simulink model "Buck_Controller_Due"  (R2020a)
settings: Solver=FixedStepAuto  StartTime=0.0  StopTime=inf  FixedStep=T  RelTol=1e-3  EnableMultiTasking=on
undefined symbols (not defined in the file): ILmax, Ki_IL, Kp_IL, Kp_Uc, T, Ubat
libraries: arduinolib x8, eeStairGenerator x1
settings Model: SILPILModeSetting=veronly  ExtModeTrigDuration=2  Creator=Nguyen Tung  LastModifiedBy=Nguyen Tung
settings OptimizationCC: StrengthReduction=on  PassReuseOutputArgsAs=Individual arguments  ZeroExternalMemoryAtStartup=off  ZeroInternalMemoryAtStartup=off  MaxStackSize=64  OptimizeBlockOrder=speed  OptimizationPriority=Speed  OptimizationCustomize=off  MultiThreadedLoops=on  EfficientTunableParamExpr=on
settings DebuggingCC: ParameterTunabilityLossMsg=error
settings HardwareCC: ProdBitPerPointer=32  ProdBitPerSizeT=32  ProdBitPerPtrDiffT=32  ProdLargestAtomicInteger=Long  ProdLargestAtomicFloat=Double  ProdWordSize=32  ProdHWDeviceType=ARM Compatible->ARM Cortex
settings SFSimCC: MATLABDynamicMemAlloc=off
settings RTWCC: SystemTargetFile=ert.tlc  HardwareBoard=Arduino Due  TLCOptions=-aInlineSetEventsForThisBaseRateFcn=TLC_FALSE -aSuppressMultiTaskScheduler=TLC_FALSE -aRateBasedStepFcn=1  TemplateMakefile=ert_default_tmf  GenerateReport=on  Toolchain=Arduino ARM  BuildConfiguration=Faster Runs
settings CodeAppCC: ForceParamTrailComments=on  IgnoreCustomStorageClasses=off  OperatorAnnotations=on  SimulinkDataObjDesc=on  SFDataObjDesc=on  InsertBlockDesc=on
settings ERTTargetCC: SupportContinuousTime=on  SupportVariableSizeSignals=on  ExtModeStaticAllocSize=20000

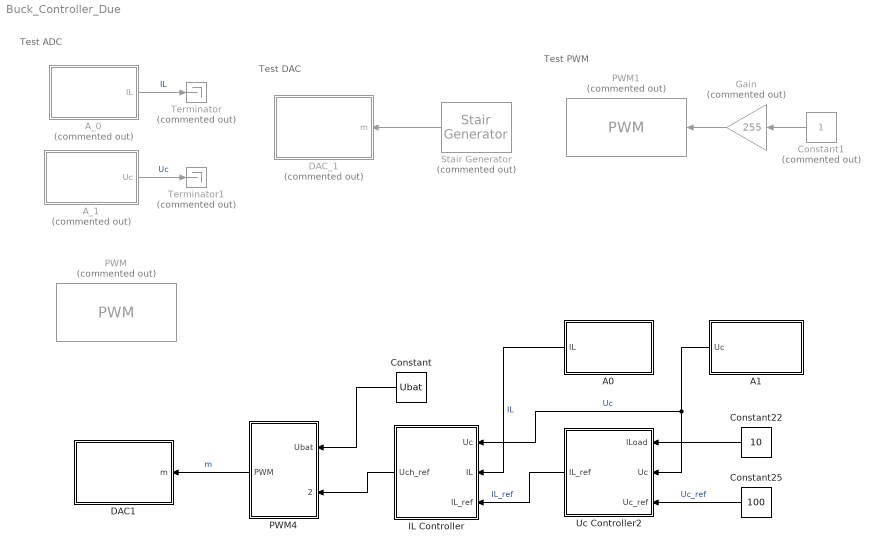
== system Buck_Controller_Due ==
  note: Test PWM
  note: Test DAC
  note: Test ADC
  A0 : Subsystem
  A1 : Subsystem
  A_0 : Subsystem  Commented=on
  A_1 : Subsystem  Commented=on
  Constant : Constant  Value=Ubat
  Constant1 : Constant  Commented=on
  Constant22 : Constant  Value=10
  Constant25 : Constant  Value=100  SampleTime=T
  DAC1 : Subsystem
  DAC_1 : Subsystem  Commented=on
  Gain : Gain  Commented=on  Gain=255
  IL Controller : Subsystem  AncestorBlock=simulink/SMC/Asservissement Correcteur IP
      mask Display: plot(0,0,100,100, [10,30,90,70,10,90],[90,10,10,90,90,10])
  PWM : arduinolib/PWM  Commented=on  pinNumber=8  frequencyType=Specify  desiredFrequency=1000  achievableFrequency=1000
  PWM1 : arduinolib/PWM  Commented=on  pinNumber=8  frequencyType=Specify  desiredFrequency=1000  achievableFrequency=1000
  PWM4 : Subsystem  AncestorBlock=simulink/SMC/Inversion EC avec mesure
      mask Display: plot(0,0,100,100,[10,30,90,70,10],[90,10,10,90,90])
  Stair Generator : eeStairGenerator/Stair Generator  Commented=on  LabelModeActiveChoice=Discrete  TimeInput=[0 2 4 6 8 10 12]  AmplitudeInput=[0 0.2 0.4 0.6 0.8 1 0]  SampleTime=T  RepeatPattern=on  OutDataTypeStr=double
      settings: SourceProductBaseCode=PS
  Terminator : Terminator  Commented=on
  Terminator1 : Terminator  Commented=on
  Uc Controller2 : Subsystem  AncestorBlock=simulink/SMC/Asservissement Correcteur IP
      mask Display: plot(0,0,100,100, [10,30,90,70,10,90],[90,10,10,90,90,10])
  wires:
  Constant25/1 -> Uc Controller2/3(Uc_ref)  "Uc_ref"
  IL Controller/1(Uch_ref) -> PWM4/2(Uch_ref)
  Uc Controller2/1(IL_ref) -> IL Controller/3(IL_ref)  "IL_ref"
  Constant22/1 -> Uc Controller2/1(ILoad)
  A_1/1(Uc) -> Terminator1/1  "Uc"
  A_0/1(IL) -> Terminator/1  "IL"
  Stair Generator/1 -> DAC_1/1(m)
  Gain/1 -> PWM1/1
  Constant1/1 -> Gain/1
  A0/1(IL) -> IL Controller/2(IL)  "IL"
  A1/1(Uc) -> IL Controller/1(Uc), Uc Controller2/2(Uc)  "Uc"
  PWM4/1(PWM) -> DAC1/1(m)  "m"
  Constant/1 -> PWM4/1(Ubat)

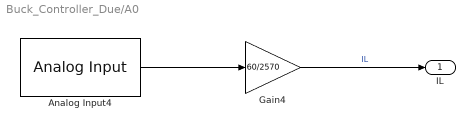
== system Buck_Controller_Due/A0 ==
  Analog Input4 : arduinolib/Analog Input  pinNumber=0  ReadResultsOnly=off  ConversionTriggerSource=Software  ExternalTriggerType=uint32( 0 )  OutputDataType=uint16  EnableConversionCompleteNotify=off  EnableOuputStatus=off  SampleTime=T  blockPlatform=arduino
  Gain4 : Gain  Gain=60/2570
  IL : Outport
  wires:
  Analog Input4/1 -> Gain4/1
  Gain4/1 -> IL/1  "IL"

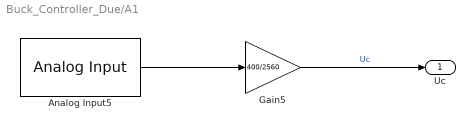
== system Buck_Controller_Due/A1 ==
  Analog Input5 : arduinolib/Analog Input  pinNumber=1  ReadResultsOnly=off  ConversionTriggerSource=Software  ExternalTriggerType=uint32( 0 )  OutputDataType=uint16  EnableConversionCompleteNotify=off  EnableOuputStatus=off  SampleTime=T  blockPlatform=arduino
  Gain5 : Gain  Gain=400/2560
  Uc : Outport
  wires:
  Analog Input5/1 -> Gain5/1
  Gain5/1 -> Uc/1  "Uc"

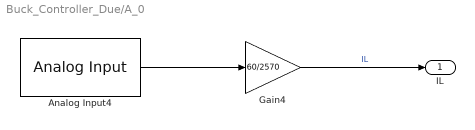
== system Buck_Controller_Due/A_0 ==
  Analog Input4 : arduinolib/Analog Input  pinNumber=0  ReadResultsOnly=off  ConversionTriggerSource=Software  ExternalTriggerType=uint32( 0 )  OutputDataType=uint16  EnableConversionCompleteNotify=off  EnableOuputStatus=off  SampleTime=T  blockPlatform=arduino
  Gain4 : Gain  Gain=60/2570
  IL : Outport
  wires:
  Analog Input4/1 -> Gain4/1
  Gain4/1 -> IL/1  "IL"

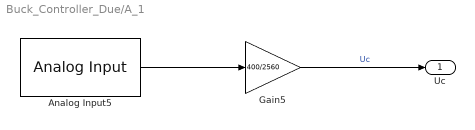
== system Buck_Controller_Due/A_1 ==
  Analog Input5 : arduinolib/Analog Input  pinNumber=1  ReadResultsOnly=off  ConversionTriggerSource=Software  ExternalTriggerType=uint32( 0 )  OutputDataType=uint16  EnableConversionCompleteNotify=off  EnableOuputStatus=off  SampleTime=T  blockPlatform=arduino
  Gain5 : Gain  Gain=400/2560
  Uc : Outport
  wires:
  Analog Input5/1 -> Gain5/1
  Gain5/1 -> Uc/1  "Uc"

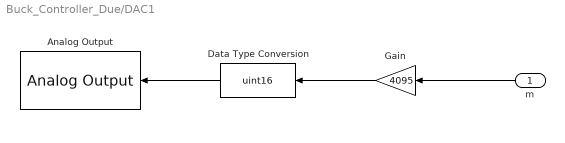
== system Buck_Controller_Due/DAC1 ==
  m : Inport
  Analog Output : arduinolib/Analog Output  DACpin=DAC1  blockPlatform=arduino
      settings: SourceProductBaseCode=ARDUINO
  Data Type Conversion : DataTypeConversion  OutDataTypeStr=uint16
  Gain : Gain  Gain=4095
  wires:
  m/1 -> Gain/1
  Gain/1 -> Data Type Conversion/1
  Data Type Conversion/1 -> Analog Output/1

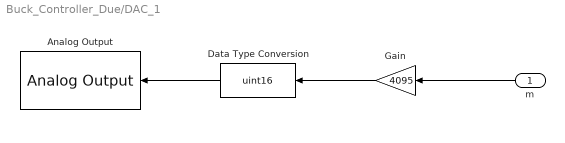
== system Buck_Controller_Due/DAC_1 ==
  m : Inport
  Analog Output : arduinolib/Analog Output  DACpin=DAC1  blockPlatform=arduino
      settings: SourceProductBaseCode=ARDUINO
  Data Type Conversion : DataTypeConversion  OutDataTypeStr=uint16
  Gain : Gain  Gain=4095
  wires:
  m/1 -> Gain/1
  Gain/1 -> Data Type Conversion/1
  Data Type Conversion/1 -> Analog Output/1

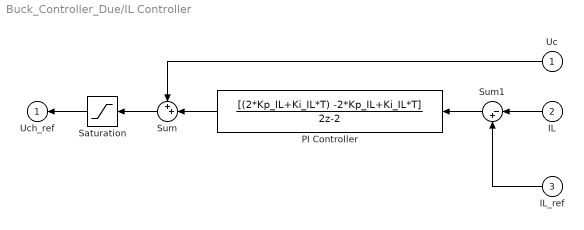
== system Buck_Controller_Due/IL Controller ==
  Uc : Inport
  IL : Inport  Port=2
  IL_ref : Inport  Port=3
  PI Controller : DiscreteTransferFcn  Numerator=[(2*Kp_IL+Ki_IL*T) -2*Kp_IL+Ki_IL*T]  Denominator=[2 -2]
  Saturation : Saturate  UpperLimit=Ubat  LowerLimit=0
  Sum : Sum  Inputs=++|
  Sum1 : Sum  Inputs=|-+
  Uch_ref : Outport  InitialOutput=0
  wires:
  Uc/1 -> Sum/1
  IL_ref/1 -> Sum1/2
  IL/1 -> Sum1/1
  Sum/1 -> Saturation/1
  Saturation/1 -> Uch_ref/1
  PI Controller/1 -> Sum/2
  Sum1/1 -> PI Controller/1

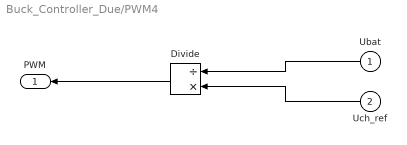
== system Buck_Controller_Due/PWM4 ==
  Ubat : Inport
  Uch_ref : Inport  Port=2
  Divide : Product  Inputs=/*
  PWM : Outport
  wires:
  Ubat/1 -> Divide/1
  Uch_ref/1 -> Divide/2
  Divide/1 -> PWM/1

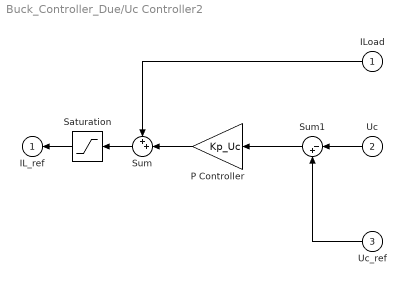
== system Buck_Controller_Due/Uc Controller2 ==
  ILoad : Inport
  Uc : Inport  Port=2
  Uc_ref : Inport  Port=3
  P Controller : Gain  Gain=Kp_Uc
  Saturation : Saturate  UpperLimit=ILmax  LowerLimit=0
  Sum : Sum  Inputs=++|
  Sum1 : Sum  Inputs=|-+
  IL_ref : Outport  InitialOutput=0
  wires:
  Uc/1 -> Sum1/1
  Uc_ref/1 -> Sum1/2
  Sum1/1 -> P Controller/1
  P Controller/1 -> Sum/2
  ILoad/1 -> Sum/1
  Sum/1 -> Saturation/1
  Saturation/1 -> IL_ref/1
